simulink model "Task_1"  (R2018b)
settings: Solver=FixedStepDiscrete  StartTime=0.0  StopTime=10.0  RelTol=1e-3
settings Model: Creator=asmaa  LastModifiedBy=asmaa
settings OptimizationCC: DefaultParameterBehavior=Inlined  EnhancedBackFolding=on  PassReuseOutputArgsAs=Individual arguments  OptimizeBlockOrder=speed  DifferentSizesBufferReuse=on  OptimizationCustomize=off
settings DebuggingCC: UnderspecifiedInitializationDetection=Classic  MergeDetectMultiDrivingBlocksExec=none  ParameterTunabilityLossMsg=error
settings ModelReferenceCC: PropagateSignalLabelsOutOfModel=off
settings SFSimCC: MATLABDynamicMemAlloc=off
settings RTWCC: SystemTargetFile=ert.tlc  GenCodeOnly=on  TemplateMakefile=ert_default_tmf  GenerateReport=on  IncludeHyperlinkInReport=on  LaunchReport=on  GenerateTraceInfo=on  GenerateTraceReport=on  GenerateTraceReportSl=on  GenerateTraceReportSf=on  GenerateTraceReportEml=on
settings CodeAppCC: ForceParamTrailComments=on  IgnoreCustomStorageClasses=off  OperatorAnnotations=on  SimulinkDataObjDesc=on  SFDataObjDesc=on  InsertBlockDesc=on
settings ERTTargetCC: TargetLangStandard=C99 (ISO)  GenerateSampleERTMain=on  InlinedParameterPlacement=NonHierarchical  ERTCustomFileTemplate=example_file_process.tlc

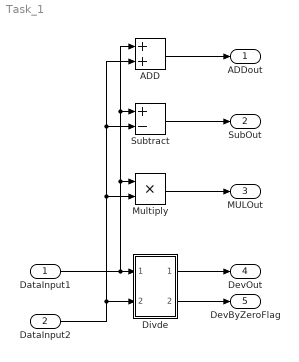
== system Task_1 ==
  "DataInput1 " : Inport
  DataInput2 : Inport  Port=2
  ADD : Sum
  Divde : Subsystem
  "Multiply " : Product
  "Subtract " : Sum  Inputs=+-
  ADDout : Outport
  "SubOut " : Outport  Port=2
  MULOut : Outport  Port=3
  DevOut : Outport  Port=4
  DevByZeroFlag : Outport  Port=5  OutDataTypeStr=boolean
  wires:
  "Subtract "/1 -> "SubOut "/1
  "Multiply "/1 -> MULOut/1
  ADD/1 -> ADDout/1
  "DataInput1 "/1 -> Divde/1(In1), "Multiply "/1, "Subtract "/1, ADD/1
  DataInput2/1 -> Divde/2(In3), ADD/2, "Subtract "/2, "Multiply "/2
  Divde/1(Out1) -> DevOut/1
  Divde/2(Out2) -> DevByZeroFlag/1

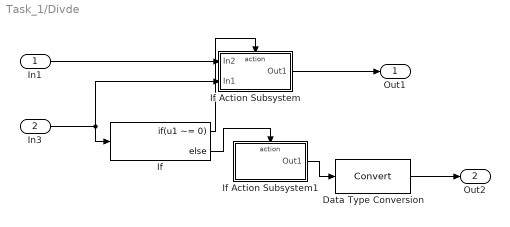
== system Task_1/Divde ==
  In1 : Inport
  In3 : Inport  Port=2
  Data Type Conversion : DataTypeConversion
  If : If  IfExpression=u1 ~= 0
  If Action Subsystem : Subsystem  TreatAsAtomicUnit=on
  If Action Subsystem1 : Subsystem  TreatAsAtomicUnit=on
  Out1 : Outport
  Out2 : Outport  Port=2  OutDataTypeStr=boolean
  wires:
  If/1 -> If Action Subsystem/Action
  In3/1 -> If/1, If Action Subsystem/2(In1)
  If/2 -> If Action Subsystem1/Action
  In1/1 -> If Action Subsystem/1(In2)
  If Action Subsystem/1(Out1) -> Out1/1
  Data Type Conversion/1 -> Out2/1
  If Action Subsystem1/1(Out1) -> Data Type Conversion/1

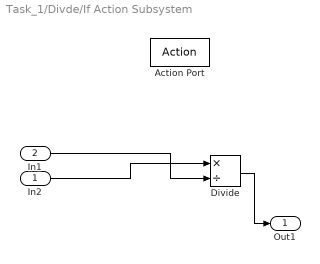
== system Task_1/Divde/If Action Subsystem ==
  In2 : Inport
  In1 : Inport  Port=2
  Action Port : ActionPort  ActionType=then
  Divide : Product  Inputs=*/
  Out1 : Outport
  wires:
  Divide/1 -> Out1/1
  In2/1 -> Divide/1
  In1/1 -> Divide/2

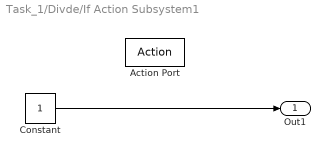
== system Task_1/Divde/If Action Subsystem1 ==
  Action Port : ActionPort  ActionType=else
  Constant : Constant
  Out1 : Outport
  wires:
  Constant/1 -> Out1/1
